simulink model "KillerWhaleModelPneumaticControl"  (R2020b)
settings: Solver=ode15s  StartTime=0.0  StopTime=10  MaxStep=0.01  RelTol=1e-3
model workspace: external: MATLAB File KillerWhaleParams.m (data not in the file)
undefined symbols (not defined in the file or in its folder): frontParams, rearParams, standParams, X, Y, Z
libraries: sm_lib x4301, nesl_utility x6
(part 3 of 66)

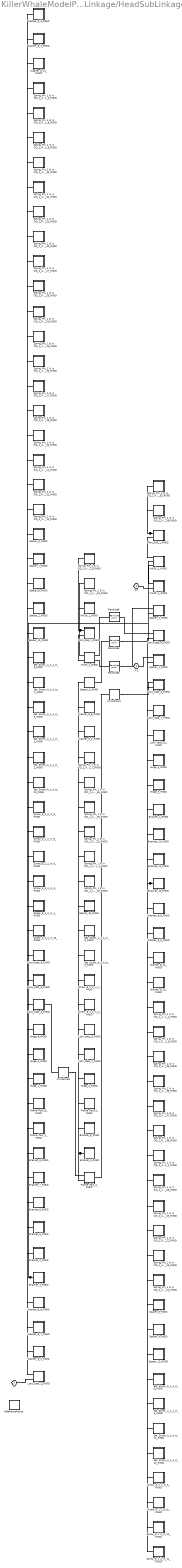
== system KillerWhaleModelPneumaticControl/HeadLinkage/HeadSubLinkage_1 ==
  Bracket_10_RIGID : Subsystem
  Bracket_11_RIGID : Subsystem
  Bracket_12_RIGID : Subsystem
  Bracket_1_RIGID : Subsystem
  Bracket_2_RIGID : Subsystem
  Bracket_3_RIGID : Subsystem
  Bracket_4_RIGID : Subsystem
  Bracket_5_RIGID : Subsystem
  Bracket_6_RIGID : Subsystem
  Bracket_7_RIGID : Subsystem
  Bracket_8_RIGID : Subsystem
  Bracket_9_RIGID : Subsystem
  Cylindrical1 : sm_lib/Joints/Cylindrical Joint  JointMode=Normal  SenseConstraintForce=off  SenseConstraintForceX=off  SenseConstraintForceY=off  SenseConstraintForceZ=off  SenseConstraintTorque=off  SenseConstraintTorqueX=off  SenseConstraintTorqueY=off  SenseConstraintTorqueZ=off  SenseTotalForce=off  SenseTotalForceX=off  SenseTotalForceY=off  SenseTotalForceZ=off  SenseTotalTorque=off  SenseTotalTorqueX=off  SenseTotalTorqueY=off  SenseTotalTorqueZ=off  CompositeWrenchDir=FollowerOnBase  CompositeWrenchFrame=BaseFrame  PzEquilibriumPosition=0  PzEquilibriumPositionUnits=m  PzSpringStiffness=0  PzSpringStiffnessUnits=N/m  PzDampingCoefficient=0  PzDampingCoefficientUnits=N/(m/s)  PzTorqueActuationMode=NoTorque  PzMotionActuationMode=ComputedMotion  PzSensePosition=off  PzSenseVelocity=off  PzSenseAcceleration=off  PzSenseTorqueForce=off  PzSenseLowerLimitTorqueForce=off  PzSenseUpperLimitTorqueForce=off  PzLowerLimitSpecify=off  PzLowerLimitBound=-1  PzLowerLimitBoundUnits=m  PzLowerLimitStiffness=1e6  PzLowerLimitStiffnessUnits=N/m  PzLowerLimitDamping=1e3  PzLowerLimitDampingUnits=N/(m/s)  PzLowerLimitTransitionRegionWidth=1e-4  PzLowerLimitTransitionRegionWidthUnits=m  PzUpperLimitSpecify=off  PzUpperLimitBound=1  PzUpperLimitBoundUnits=m  PzUpperLimitStiffness=1e6  PzUpperLimitStiffnessUnits=N/m  PzUpperLimitDamping=1e3  PzUpperLimitDampingUnits=N/(m/s)  PzUpperLimitTransitionRegionWidth=1e-4  PzUpperLimitTransitionRegionWidthUnits=m  PzPositionTargetSpecify=off  PzPositionTargetPriority=High  PzPositionTargetValue=0  PzPositionTargetValueUnits=m  PzVelocityTargetSpecify=off  PzVelocityTargetPriority=High  PzVelocityTargetValue=0  PzVelocityTargetValueUnits=m/s  RzEquilibriumPosition=0  RzEquilibriumPositionUnits=deg  RzSpringStiffness=0  RzSpringStiffnessUnits=N*m/deg  RzDampingCoefficient=0  RzDampingCoefficientUnits=N*m/(deg/s)  RzTorqueActuationMode=NoTorque  RzMotionActuationMode=ComputedMotion  RzSensePosition=off  RzSenseVelocity=off  RzSenseAcceleration=off  RzSenseTorqueForce=off  RzSenseLowerLimitTorqueForce=off  RzSenseUpperLimitTorqueForce=off  RzLowerLimitSpecify=off  RzLowerLimitBound=-90  RzLowerLimitBoundUnits=deg  RzLowerLimitStiffness=1e4  RzLowerLimitStiffnessUnits=N*m/deg  RzLowerLimitDamping=10  RzLowerLimitDampingUnits=N*m/(deg/s)  RzLowerLimitTransitionRegionWidth=0.1  RzLowerLimitTransitionRegionWidthUnits=deg  RzUpperLimitSpecify=off  RzUpperLimitBound=90  RzUpperLimitBoundUnits=deg  RzUpperLimitStiffness=1e4  RzUpperLimitStiffnessUnits=N*m/deg  RzUpperLimitDamping=10  RzUpperLimitDampingUnits=N*m/(deg/s)  RzUpperLimitTransitionRegionWidth=0.1  RzUpperLimitTransitionRegionWidthUnits=deg  RzPositionTargetSpecify=off  RzPositionTargetPriority=High  RzPositionTargetValue=0  RzPositionTargetValueUnits=deg  RzVelocityTargetSpecify=off  RzVelocityTargetPriority=High  RzVelocityTargetValue=0  RzVelocityTargetValueUnits=deg/s
  Cylindrical2 : sm_lib/Joints/Cylindrical Joint  JointMode=Normal  SenseConstraintForce=off  SenseConstraintForceX=off  SenseConstraintForceY=off  SenseConstraintForceZ=off  SenseConstraintTorque=off  SenseConstraintTorqueX=off  SenseConstraintTorqueY=off  SenseConstraintTorqueZ=off  SenseTotalForce=off  SenseTotalForceX=off  SenseTotalForceY=off  SenseTotalForceZ=off  SenseTotalTorque=off  SenseTotalTorqueX=off  SenseTotalTorqueY=off  SenseTotalTorqueZ=off  CompositeWrenchDir=FollowerOnBase  CompositeWrenchFrame=BaseFrame  PzEquilibriumPosition=0  PzEquilibriumPositionUnits=m  PzSpringStiffness=0  PzSpringStiffnessUnits=N/m  PzDampingCoefficient=0  PzDampingCoefficientUnits=N/(m/s)  PzTorqueActuationMode=NoTorque  PzMotionActuationMode=ComputedMotion  PzSensePosition=off  PzSenseVelocity=off  PzSenseAcceleration=off  PzSenseTorqueForce=off  PzSenseLowerLimitTorqueForce=off  PzSenseUpperLimitTorqueForce=off  PzLowerLimitSpecify=off  PzLowerLimitBound=-1  PzLowerLimitBoundUnits=m  PzLowerLimitStiffness=1e6  PzLowerLimitStiffnessUnits=N/m  PzLowerLimitDamping=1e3  PzLowerLimitDampingUnits=N/(m/s)  PzLowerLimitTransitionRegionWidth=1e-4  PzLowerLimitTransitionRegionWidthUnits=m  PzUpperLimitSpecify=off  PzUpperLimitBound=1  PzUpperLimitBoundUnits=m  PzUpperLimitStiffness=1e6  PzUpperLimitStiffnessUnits=N/m  PzUpperLimitDamping=1e3  PzUpperLimitDampingUnits=N/(m/s)  PzUpperLimitTransitionRegionWidth=1e-4  PzUpperLimitTransitionRegionWidthUnits=m  PzPositionTargetSpecify=off  PzPositionTargetPriority=High  PzPositionTargetValue=0  PzPositionTargetValueUnits=m  PzVelocityTargetSpecify=off  PzVelocityTargetPriority=High  PzVelocityTargetValue=0  PzVelocityTargetValueUnits=m/s  RzEquilibriumPosition=0  RzEquilibriumPositionUnits=deg  RzSpringStiffness=0  RzSpringStiffnessUnits=N*m/deg  RzDampingCoefficient=0  RzDampingCoefficientUnits=N*m/(deg/s)  RzTorqueActuationMode=NoTorque  RzMotionActuationMode=ComputedMotion  RzSensePosition=off  RzSenseVelocity=off  RzSenseAcceleration=off  RzSenseTorqueForce=off  RzSenseLowerLimitTorqueForce=off  RzSenseUpperLimitTorqueForce=off  RzLowerLimitSpecify=off  RzLowerLimitBound=-90  RzLowerLimitBoundUnits=deg  RzLowerLimitStiffness=1e4  RzLowerLimitStiffnessUnits=N*m/deg  RzLowerLimitDamping=10  RzLowerLimitDampingUnits=N*m/(deg/s)  RzLowerLimitTransitionRegionWidth=0.1  RzLowerLimitTransitionRegionWidthUnits=deg  RzUpperLimitSpecify=off  RzUpperLimitBound=90  RzUpperLimitBoundUnits=deg  RzUpperLimitStiffness=1e4  RzUpperLimitStiffnessUnits=N*m/deg  RzUpperLimitDamping=10  RzUpperLimitDampingUnits=N*m/(deg/s)  RzUpperLimitTransitionRegionWidth=0.1  RzUpperLimitTransitionRegionWidthUnits=deg  RzPositionTargetSpecify=off  RzPositionTargetPriority=High  RzPositionTargetValue=0  RzPositionTargetValueUnits=deg  RzVelocityTargetSpecify=off  RzVelocityTargetPriority=High  RzVelocityTargetValue=0  RzVelocityTargetValueUnits=deg/s
  Frame_Part_1_RIGID : Subsystem
  Frame_Part_2_RIGID : Subsystem
  Frame_Part_3_RIGID : Subsystem
  Frame_Part_4_RIGID : Subsystem
  Hinge_1_RIGID : Subsystem
  Hinge_2_RIGID : Subsystem
  Hinge_3_RIGID : Subsystem
  Hinge_4_RIGID : Subsystem
  Hinge_5_RIGID : Subsystem
  Hinge_6_RIGID : Subsystem
  Lock_tabs_10_RIGID : Subsystem
  Lock_tabs_1_RIGID : Subsystem
  Lock_tabs_2_RIGID : Subsystem
  Lock_tabs_3_RIGID : Subsystem
  Lock_tabs_4_RIGID : Subsystem
  Lock_tabs_5_RIGID : Subsystem
  Lock_tabs_6_RIGID : Subsystem
  Lock_tabs_7_RIGID : Subsystem
  Lock_tabs_8_RIGID : Subsystem
  Lock_tabs_9_RIGID : Subsystem
  Part_843_1_RIGID : Subsystem
  Part_844_1_RIGID : Subsystem
  ReferenceFrame : sm_lib/Frames and Transforms/Reference Frame
  Revolute3 : sm_lib/Joints/Revolute Joint  JointMode=Normal  SenseConstraintForce=off  SenseConstraintForceX=off  SenseConstraintForceY=off  SenseConstraintForceZ=off  SenseConstraintTorque=off  SenseConstraintTorqueX=off  SenseConstraintTorqueY=off  SenseConstraintTorqueZ=off  SenseTotalForce=off  SenseTotalForceX=off  SenseTotalForceY=off  SenseTotalForceZ=off  SenseTotalTorque=off  SenseTotalTorqueX=off  SenseTotalTorqueY=off  SenseTotalTorqueZ=off  CompositeWrenchDir=FollowerOnBase  CompositeWrenchFrame=BaseFrame  EquilibriumPosition=0  EquilibriumPositionUnits=deg  SpringStiffness=0  SpringStiffnessUnits=N*m/deg  DampingCoefficient=0  DampingCoefficientUnits=N*m/(deg/s)  TorqueActuationMode=NoTorque  MotionActuationMode=ComputedMotion  SensePosition=off  SenseVelocity=off  SenseAcceleration=off  SenseTorqueForce=off  SenseLowerLimitTorqueForce=off  SenseUpperLimitTorqueForce=off  LowerLimitSpecify=off  LowerLimitBound=-90  LowerLimitBoundUnits=deg  LowerLimitStiffness=1e4  LowerLimitStiffnessUnits=N*m/deg  LowerLimitDamping=10  LowerLimitDampingUnits=N*m/(deg/s)  LowerLimitTransitionRegionWidth=0.1  LowerLimitTransitionRegionWidthUnits=deg  UpperLimitSpecify=off  UpperLimitBound=90  UpperLimitBoundUnits=deg  UpperLimitStiffness=1e4  UpperLimitStiffnessUnits=N*m/deg  UpperLimitDamping=10  UpperLimitDampingUnits=N*m/(deg/s)  UpperLimitTransitionRegionWidth=0.1  UpperLimitTransitionRegionWidthUnits=deg  PositionTargetSpecify=on  PositionTargetPriority=Low  PositionTargetValue=frontParams.RevoluteJoint(3).Rz.Pos  PositionTargetValueUnits=deg  VelocityTargetSpecify=off  VelocityTargetPriority=High  VelocityTargetValue=0  VelocityTargetValueUnits=deg/s
  Revolute5 : sm_lib/Joints/Revolute Joint  JointMode=Normal  SenseConstraintForce=off  SenseConstraintForceX=off  SenseConstraintForceY=off  SenseConstraintForceZ=off  SenseConstraintTorque=off  SenseConstraintTorqueX=off  SenseConstraintTorqueY=off  SenseConstraintTorqueZ=off  SenseTotalForce=off  SenseTotalForceX=off  SenseTotalForceY=off  SenseTotalForceZ=off  SenseTotalTorque=off  SenseTotalTorqueX=off  SenseTotalTorqueY=off  SenseTotalTorqueZ=off  CompositeWrenchDir=FollowerOnBase  CompositeWrenchFrame=BaseFrame  EquilibriumPosition=0  EquilibriumPositionUnits=deg  SpringStiffness=0  SpringStiffnessUnits=N*m/deg  DampingCoefficient=0  DampingCoefficientUnits=N*m/(deg/s)  TorqueActuationMode=NoTorque  MotionActuationMode=ComputedMotion  SensePosition=off  SenseVelocity=off  SenseAcceleration=off  SenseTorqueForce=off  SenseLowerLimitTorqueForce=off  SenseUpperLimitTorqueForce=off  LowerLimitSpecify=off  LowerLimitBound=-90  LowerLimitBoundUnits=deg  LowerLimitStiffness=1e4  LowerLimitStiffnessUnits=N*m/deg  LowerLimitDamping=10  LowerLimitDampingUnits=N*m/(deg/s)  LowerLimitTransitionRegionWidth=0.1  LowerLimitTransitionRegionWidthUnits=deg  UpperLimitSpecify=off  UpperLimitBound=90  UpperLimitBoundUnits=deg  UpperLimitStiffness=1e4  UpperLimitStiffnessUnits=N*m/deg  UpperLimitDamping=10  UpperLimitDampingUnits=N*m/(deg/s)  UpperLimitTransitionRegionWidth=0.1  UpperLimitTransitionRegionWidthUnits=deg  PositionTargetSpecify=on  PositionTargetPriority=Low  PositionTargetValue=frontParams.RevoluteJoint(1).Rz.Pos  PositionTargetValueUnits=deg  VelocityTargetSpecify=off  VelocityTargetPriority=High  VelocityTargetValue=0  VelocityTargetValueUnits=deg/s
  Revolute6 : sm_lib/Joints/Revolute Joint  JointMode=Normal  SenseConstraintForce=off  SenseConstraintForceX=off  SenseConstraintForceY=off  SenseConstraintForceZ=off  SenseConstraintTorque=off  SenseConstraintTorqueX=off  SenseConstraintTorqueY=off  SenseConstraintTorqueZ=off  SenseTotalForce=off  SenseTotalForceX=off  SenseTotalForceY=off  SenseTotalForceZ=off  SenseTotalTorque=off  SenseTotalTorqueX=off  SenseTotalTorqueY=off  SenseTotalTorqueZ=off  CompositeWrenchDir=FollowerOnBase  CompositeWrenchFrame=BaseFrame  EquilibriumPosition=0  EquilibriumPositionUnits=deg  SpringStiffness=0  SpringStiffnessUnits=N*m/deg  DampingCoefficient=0  DampingCoefficientUnits=N*m/(deg/s)  TorqueActuationMode=NoTorque  MotionActuationMode=ComputedMotion  SensePosition=off  SenseVelocity=off  SenseAcceleration=off  SenseTorqueForce=off  SenseLowerLimitTorqueForce=off  SenseUpperLimitTorqueForce=off  LowerLimitSpecify=off  LowerLimitBound=-90  LowerLimitBoundUnits=deg  LowerLimitStiffness=1e4  LowerLimitStiffnessUnits=N*m/deg  LowerLimitDamping=10  LowerLimitDampingUnits=N*m/(deg/s)  LowerLimitTransitionRegionWidth=0.1  LowerLimitTransitionRegionWidthUnits=deg  UpperLimitSpecify=off  UpperLimitBound=90  UpperLimitBoundUnits=deg  UpperLimitStiffness=1e4  UpperLimitStiffnessUnits=N*m/deg  UpperLimitDamping=10  UpperLimitDampingUnits=N*m/(deg/s)  UpperLimitTransitionRegionWidth=0.1  UpperLimitTransitionRegionWidthUnits=deg  PositionTargetSpecify=on  PositionTargetPriority=Low  PositionTargetValue=frontParams.RevoluteJoint(2).Rz.Pos  PositionTargetValueUnits=deg  VelocityTargetSpecify=off  VelocityTargetPriority=High  VelocityTargetValue=0  VelocityTargetValueUnits=deg/s
  Screw_8_1_2_in_10_RIGID : Subsystem
  Screw_8_1_2_in_11_RIGID : Subsystem
  Screw_8_1_2_in_12_RIGID : Subsystem
  Screw_8_1_2_in_1_RIGID : Subsystem
  Screw_8_1_2_in_2_RIGID : Subsystem
  Screw_8_1_2_in_3_RIGID : Subsystem
  Screw_8_1_2_in_4_RIGID : Subsystem
  Screw_8_1_2_in_5_RIGID : Subsystem
  Screw_8_1_2_in_6_RIGID : Subsystem
  Screw_8_1_2_in_7_RIGID : Subsystem
  Screw_8_1_2_in_8_RIGID : Subsystem
  Screw_8_1_2_in_9_RIGID : Subsystem
  Set_Screw_4_1_4_in_10_RIGID : Subsystem
  Set_Screw_4_1_4_in_11_RIGID : Subsystem
  Set_Screw_4_1_4_in_12_RIGID : Subsystem
  Set_Screw_4_1_4_in_1_RIGID : Subsystem
  Set_Screw_4_1_4_in_2_RIGID : Subsystem
  Set_Screw_4_1_4_in_3_RIGID : Subsystem
  Set_Screw_4_1_4_in_4_RIGID : Subsystem
  Set_Screw_4_1_4_in_5_RIGID : Subsystem
  Set_Screw_4_1_4_in_6_RIGID : Subsystem
  Set_Screw_4_1_4_in_7_RIGID : Subsystem
  Set_Screw_4_1_4_in_8_RIGID : Subsystem
  Set_Screw_4_1_4_in_9_RIGID : Subsystem
  Spacer_10_RIGID : Subsystem
  Spacer_11_RIGID : Subsystem
  Spacer_12_RIGID : Subsystem
  Spacer_1_RIGID : Subsystem
  Spacer_2_RIGID : Subsystem
  Spacer_3_RIGID : Subsystem
  Spacer_4_RIGID : Subsystem
  Spacer_5_RIGID : Subsystem
  Spacer_6_RIGID : Subsystem
  Spacer_7_RIGID : Subsystem
  Spacer_8_RIGID : Subsystem
  Spacer_9_RIGID : Subsystem
  Spring_Pin_1_8_in_OD_1_4_in_L_10_RIGID : Subsystem
  Spring_Pin_1_8_in_OD_1_4_in_L_11_RIGID : Subsystem
  Spring_Pin_1_8_in_OD_1_4_in_L_12_RIGID : Subsystem
  Spring_Pin_1_8_in_OD_1_4_in_L_13_RIGID : Subsystem
  Spring_Pin_1_8_in_OD_1_4_in_L_14_RIGID : Subsystem
  Spring_Pin_1_8_in_OD_1_4_in_L_15_RIGID : Subsystem
  Spring_Pin_1_8_in_OD_1_4_in_L_16_RIGID : Subsystem
  Spring_Pin_1_8_in_OD_1_4_in_L_17_RIGID : Subsystem
  Spring_Pin_1_8_in_OD_1_4_in_L_18_RIGID : Subsystem
  Spring_Pin_1_8_in_OD_1_4_in_L_19_RIGID : Subsystem
  Spring_Pin_1_8_in_OD_1_4_in_L_1_RIGID : Subsystem
  Spring_Pin_1_8_in_OD_1_4_in_L_20_RIGID : Subsystem
  Spring_Pin_1_8_in_OD_1_4_in_L_21_RIGID : Subsystem
  Spring_Pin_1_8_in_OD_1_4_in_L_22_RIGID : Subsystem
  Spring_Pin_1_8_in_OD_1_4_in_L_23_RIGID : Subsystem
  Spring_Pin_1_8_in_OD_1_4_in_L_24_RIGID : Subsystem
  Spring_Pin_1_8_in_OD_1_4_in_L_25_RIGID : Subsystem
  Spring_Pin_1_8_in_OD_1_4_in_L_26_RIGID : Subsystem
  Spring_Pin_1_8_in_OD_1_4_in_L_27_RIGID : Subsystem
  Spring_Pin_1_8_in_OD_1_4_in_L_28_RIGID : Subsystem
  Spring_Pin_1_8_in_OD_1_4_in_L_29_RIGID : Subsystem
  Spring_Pin_1_8_in_OD_1_4_in_L_2_RIGID : Subsystem
  Spring_Pin_1_8_in_OD_1_4_in_L_30_RIGID : Subsystem
  Spring_Pin_1_8_in_OD_1_4_in_L_31_RIGID : Subsystem
  Spring_Pin_1_8_in_OD_1_4_in_L_32_RIGID : Subsystem
  Spring_Pin_1_8_in_OD_1_4_in_L_33_RIGID : Subsystem
  Spring_Pin_1_8_in_OD_1_4_in_L_34_RIGID : Subsystem
  Spring_Pin_1_8_in_OD_1_4_in_L_35_RIGID : Subsystem
  Spring_Pin_1_8_in_OD_1_4_in_L_36_RIGID : Subsystem
  Spring_Pin_1_8_in_OD_1_4_in_L_37_RIGID : Subsystem
  Spring_Pin_1_8_in_OD_1_4_in_L_38_RIGID : Subsystem
  Spring_Pin_1_8_in_OD_1_4_in_L_39_RIGID : Subsystem
  Spring_Pin_1_8_in_OD_1_4_in_L_3_RIGID : Subsystem
  Spring_Pin_1_8_in_OD_1_4_in_L_40_RIGID : Subsystem
  Spring_Pin_1_8_in_OD_1_4_in_L_4_RIGID : Subsystem
  Spring_Pin_1_8_in_OD_1_4_in_L_5_RIGID : Subsystem
  Spring_Pin_1_8_in_OD_1_4_in_L_6_RIGID : Subsystem
  Spring_Pin_1_8_in_OD_1_4_in_L_7_RIGID : Subsystem
  Spring_Pin_1_8_in_OD_1_4_in_L_8_RIGID : Subsystem
  Spring_Pin_1_8_in_OD_1_4_in_L_9_RIGID : Subsystem
  Washer_8_10_RIGID : Subsystem
  Washer_8_11_RIGID : Subsystem
  Washer_8_12_RIGID : Subsystem
  Washer_8_1_RIGID : Subsystem
  Washer_8_2_RIGID : Subsystem
  Washer_8_3_RIGID : Subsystem
  Washer_8_4_RIGID : Subsystem
  Washer_8_5_RIGID : Subsystem
  Washer_8_6_RIGID : Subsystem
  Washer_8_7_RIGID : Subsystem
  Washer_8_8_RIGID : Subsystem
  Washer_8_9_RIGID : Subsystem
  link1fl_1_RIGID : Subsystem
  link1fr_1_RIGID : Subsystem
  link2fl_1_RIGID : Subsystem
  link2fr_1_RIGID : Subsystem
  F2 : PMIOPort  Side=Left
  F1 : PMIOPort  Port=2  Side=Left
  F : PMIOPort  Port=3  Side=Right
  connections:
  Bracket_1_RIGID/LConn1 -- Bracket_2_RIGID/LConn1 -- Bracket_5_RIGID/LConn1 -- Bracket_6_RIGID/LConn1 -- Bracket_7_RIGID/LConn1 -- Bracket_9_RIGID/LConn1 -- Frame_Part_1_RIGID/LConn1 -- Frame_Part_3_RIGID/LConn1 -- Hinge_1_RIGID/LConn1 -- Hinge_5_RIGID/LConn1 -- Hinge_6_RIGID/LConn1 -- Lock_tabs_1_RIGID/LConn1 -- Lock_tabs_3_RIGID/LConn1 -- Lock_tabs_8_RIGID/LConn1 -- Lock_tabs_9_RIGID/LConn1 -- Screw_8_1_2_in_10_RIGID/LConn1 -- Screw_8_1_2_in_1_RIGID/LConn1 -- Screw_8_1_2_in_3_RIGID/LConn1 -- Screw_8_1_2_in_4_RIGID/LConn1 -- Screw_8_1_2_in_8_RIGID/LConn1 -- Screw_8_1_2_in_9_RIGID/LConn1 -- Set_Screw_4_1_4_in_12_RIGID/LConn1 -- Set_Screw_4_1_4_in_1_RIGID/LConn1 -- Set_Screw_4_1_4_in_2_RIGID/LConn1 -- Set_Screw_4_1_4_in_6_RIGID/LConn1 -- Set_Screw_4_1_4_in_7_RIGID/LConn1 -- Set_Screw_4_1_4_in_8_RIGID/LConn1 -- Spacer_11_RIGID/LConn1 -- Spacer_2_RIGID/LConn1 -- Spacer_5_RIGID/LConn2 -- Spacer_6_RIGID/LConn1 -- Spacer_7_RIGID/LConn1 -- Spacer_9_RIGID/LConn1 -- Spring_Pin_1_8_in_OD_1_4_in_L_11_RIGID/LConn1 -- Spring_Pin_1_8_in_OD_1_4_in_L_12_RIGID/LConn1 -- Spring_Pin_1_8_in_OD_1_4_in_L_14_RIGID/LConn1 -- Spring_Pin_1_8_in_OD_1_4_in_L_15_RIGID/LConn1 -- Spring_Pin_1_8_in_OD_1_4_in_L_16_RIGID/LConn1 -- Spring_Pin_1_8_in_OD_1_4_in_L_17_RIGID/LConn1 -- Spring_Pin_1_8_in_OD_1_4_in_L_20_RIGID/LConn1 -- Spring_Pin_1_8_in_OD_1_4_in_L_23_RIGID/LConn1 -- Spring_Pin_1_8_in_OD_1_4_in_L_24_RIGID/LConn1 -- Spring_Pin_1_8_in_OD_1_4_in_L_26_RIGID/LConn1 -- Spring_Pin_1_8_in_OD_1_4_in_L_27_RIGID/LConn1 -- Spring_Pin_1_8_in_OD_1_4_in_L_30_RIGID/LConn1 -- Spring_Pin_1_8_in_OD_1_4_in_L_31_RIGID/LConn1 -- Spring_Pin_1_8_in_OD_1_4_in_L_32_RIGID/LConn1 -- Spring_Pin_1_8_in_OD_1_4_in_L_40_RIGID/LConn1 -- Spring_Pin_1_8_in_OD_1_4_in_L_6_RIGID/LConn1 -- Spring_Pin_1_8_in_OD_1_4_in_L_8_RIGID/LConn1 -- Spring_Pin_1_8_in_OD_1_4_in_L_9_RIGID/LConn1 -- Washer_8_11_RIGID/LConn1 -- Washer_8_1_RIGID/LConn1 -- Washer_8_3_RIGID/LConn1 -- Washer_8_4_RIGID/LConn1 -- Washer_8_7_RIGID/LConn1 -- Washer_8_9_RIGID/LConn1
  Bracket_10_RIGID/LConn1 -- Bracket_11_RIGID/LConn1 -- Bracket_12_RIGID/LConn1 -- Bracket_4_RIGID/LConn1 -- Hinge_3_RIGID/LConn1 -- Hinge_4_RIGID/LConn1 -- Lock_tabs_10_RIGID/LConn1 -- Lock_tabs_4_RIGID/LConn2 -- Lock_tabs_5_RIGID/LConn2 -- Lock_tabs_7_RIGID/LConn1 -- Screw_8_1_2_in_11_RIGID/LConn1 -- Screw_8_1_2_in_12_RIGID/LConn1 -- Screw_8_1_2_in_5_RIGID/LConn1 -- Screw_8_1_2_in_6_RIGID/LConn1 -- Set_Screw_4_1_4_in_10_RIGID/LConn1 -- Set_Screw_4_1_4_in_11_RIGID/LConn1 -- Set_Screw_4_1_4_in_4_RIGID/LConn1 -- Set_Screw_4_1_4_in_5_RIGID/LConn1 -- Spacer_12_RIGID/LConn1 -- Spacer_1_RIGID/LConn2 -- Spacer_4_RIGID/LConn1 -- Spacer_8_RIGID/LConn1 -- Spring_Pin_1_8_in_OD_1_4_in_L_10_RIGID/LConn1 -- Spring_Pin_1_8_in_OD_1_4_in_L_13_RIGID/LConn1 -- Spring_Pin_1_8_in_OD_1_4_in_L_22_RIGID/LConn1 -- Spring_Pin_1_8_in_OD_1_4_in_L_25_RIGID/LConn1 -- Spring_Pin_1_8_in_OD_1_4_in_L_28_RIGID/LConn1 -- Spring_Pin_1_8_in_OD_1_4_in_L_2_RIGID/LConn1 -- Spring_Pin_1_8_in_OD_1_4_in_L_36_RIGID/LConn1 -- Spring_Pin_1_8_in_OD_1_4_in_L_37_RIGID/LConn1 -- Spring_Pin_1_8_in_OD_1_4_in_L_38_RIGID/LConn1 -- Spring_Pin_1_8_in_OD_1_4_in_L_39_RIGID/LConn1 -- Spring_Pin_1_8_in_OD_1_4_in_L_3_RIGID/LConn1 -- Spring_Pin_1_8_in_OD_1_4_in_L_4_RIGID/LConn1 -- Washer_8_10_RIGID/LConn1 -- Washer_8_12_RIGID/LConn1 -- Washer_8_5_RIGID/LConn1 -- Washer_8_6_RIGID/LConn1
  Revolute5/RConn1 -- Spacer_5_RIGID/LConn1
  Revolute6/LConn1 -- link2fl_1_RIGID/RConn1
  Lock_tabs_4_RIGID/LConn1 -- Revolute6/RConn1
  Cylindrical2/LConn1 -- Lock_tabs_3_RIGID/RConn1
  Cylindrical2/RConn1 -- Frame_Part_2_RIGID/LConn1
  Part_844_1_RIGID/LConn2 -- link2fl_1_RIGID/LConn2
  Revolute3/LConn1 -- Spacer_3_RIGID/RConn1
  Revolute3/RConn1 -- link1fl_1_RIGID/LConn3
  Part_843_1_RIGID/LConn2 -- link1fl_1_RIGID/LConn1
  Lock_tabs_1_RIGID/LConn2 -- F/RConn1
  link1fl_1_RIGID/LConn2 -- link1fr_1_RIGID/LConn1
  Spacer_1_RIGID/LConn1 -- F1/RConn1
  link1fr_1_RIGID/LConn2 -- F2/RConn1
  Part_843_1_RIGID/LConn1 -- Spring_Pin_1_8_in_OD_1_4_in_L_18_RIGID/LConn1 -- Spring_Pin_1_8_in_OD_1_4_in_L_33_RIGID/LConn1
  link2fl_1_RIGID/LConn1 -- link2fr_1_RIGID/LConn1
  Bracket_3_RIGID/LConn1 -- Bracket_8_RIGID/LConn1 -- Frame_Part_2_RIGID/LConn2 -- Frame_Part_4_RIGID/LConn1 -- Hinge_2_RIGID/LConn1 -- Lock_tabs_2_RIGID/LConn1 -- Lock_tabs_6_RIGID/LConn1 -- Screw_8_1_2_in_2_RIGID/LConn1 -- Screw_8_1_2_in_7_RIGID/LConn1 -- Set_Screw_4_1_4_in_3_RIGID/LConn1 -- Set_Screw_4_1_4_in_9_RIGID/LConn1 -- Spacer_10_RIGID/LConn1 -- Spacer_3_RIGID/LConn1 -- Spring_Pin_1_8_in_OD_1_4_in_L_19_RIGID/LConn1 -- Spring_Pin_1_8_in_OD_1_4_in_L_1_RIGID/LConn1 -- Spring_Pin_1_8_in_OD_1_4_in_L_21_RIGID/LConn1 -- Spring_Pin_1_8_in_OD_1_4_in_L_29_RIGID/LConn1 -- Spring_Pin_1_8_in_OD_1_4_in_L_35_RIGID/LConn1 -- Spring_Pin_1_8_in_OD_1_4_in_L_7_RIGID/LConn1 -- Washer_8_2_RIGID/LConn1 -- Washer_8_8_RIGID/LConn1
  Part_844_1_RIGID/LConn1 -- Spring_Pin_1_8_in_OD_1_4_in_L_34_RIGID/LConn1 -- Spring_Pin_1_8_in_OD_1_4_in_L_5_RIGID/LConn1
  Cylindrical1/LConn1 -- Frame_Part_2_RIGID/RConn1
  Cylindrical1/RConn1 -- Lock_tabs_5_RIGID/LConn1
  Revolute5/LConn1 -- link2fl_1_RIGID/RConn2

== system KillerWhaleModelPneumaticControl/HeadLinkage/Head_Actuator_1 ==
  Part_10_1_RIGID : Subsystem
  Part_11_1_RIGID : Subsystem
  Part_12_1_RIGID : Subsystem
  Part_13_1_RIGID : Subsystem
  Part_1_1_RIGID : Subsystem
  Part_2_1_RIGID : Subsystem
  Part_3_1_RIGID : Subsystem
  Part_4_1_RIGID : Subsystem
  Part_5_1_RIGID : Subsystem
  Part_6_1_RIGID : Subsystem
  Part_7_1_RIGID : Subsystem
  Part_8_1_RIGID : Subsystem
  Part_9_1_RIGID : Subsystem
  ReferenceFrame : sm_lib/Frames and Transforms/Reference Frame
  Slider1 : sm_lib/Joints/Prismatic Joint  JointMode=Normal  SenseConstraintForce=off  SenseConstraintForceX=off  SenseConstraintForceY=off  SenseConstraintForceZ=off  SenseConstraintTorque=off  SenseConstraintTorqueX=off  SenseConstraintTorqueY=off  SenseConstraintTorqueZ=off  SenseTotalForce=off  SenseTotalForceX=off  SenseTotalForceY=off  SenseTotalForceZ=off  SenseTotalTorque=off  SenseTotalTorqueX=off  SenseTotalTorqueY=off  SenseTotalTorqueZ=off  CompositeWrenchDir=FollowerOnBase  CompositeWrenchFrame=BaseFrame  EquilibriumPosition=0  EquilibriumPositionUnits=m  SpringStiffness=0  SpringStiffnessUnits=N/m  DampingCoefficient=0  DampingCoefficientUnits=N/(m/s)  TorqueActuationMode=ComputedTorque  MotionActuationMode=InputMotion  SensePosition=off  SenseVelocity=off  SenseAcceleration=off  SenseTorqueForce=off  SenseLowerLimitTorqueForce=off  SenseUpperLimitTorqueForce=off  LowerLimitSpecify=off  LowerLimitBound=-1  LowerLimitBoundUnits=m  LowerLimitStiffness=1e6  LowerLimitStiffnessUnits=N/m  LowerLimitDamping=1e3  LowerLimitDampingUnits=N/(m/s)  LowerLimitTransitionRegionWidth=1e-4  LowerLimitTransitionRegionWidthUnits=m  UpperLimitSpecify=off  UpperLimitBound=1  UpperLimitBoundUnits=m  UpperLimitStiffness=1e6  UpperLimitStiffnessUnits=N/m  UpperLimitDamping=1e3  UpperLimitDampingUnits=N/(m/s)  UpperLimitTransitionRegionWidth=1e-4  UpperLimitTransitionRegionWidthUnits=m  PositionTargetSpecify=on  PositionTargetPriority=Low  PositionTargetValue=frontParams.PrismaticJoint(2).Pz.Pos  PositionTargetValueUnits=in  VelocityTargetSpecify=off  VelocityTargetPriority=High  VelocityTargetValue=0  VelocityTargetValueUnits=m/s
  Transform : sm_lib/Frames and Transforms/Rigid Transform  TranslationMethod=Cartesian  TranslationStandardOffset=0  TranslationLengthUnit=in  TranslationStandardAxis=+Z  TranslationCartesianOffset=frontParams.RigidTransform(421).translation  TranslationROffset=0  TranslationROffsetUnits=m  TranslationZOffset=0  TranslationZOffsetUnits=m  TranslationThetaOffset=0  TranslationThetaOffsetUnits=deg  RotationMethod=ArbitraryAxis  RotationAngleUnits=rad  RotationStandardAxis=+Z  RotationAngle=frontParams.RigidTransform(421).angle  RotationArbitraryAxis=frontParams.RigidTransform(421).axis  FollAlignAxisA=+X  BaseAlignAxisA=+Y  FollAlignAxisB=+Y  BaseAlignAxisB=+Z  RotationSequenceAxes=FollowerAxes  RotationSequence=XYX  RotationSequenceAngles=[0 0 0]  RotationSequenceAnglesUnits=deg  RotationMatrix=[1 0 0; 0 1 0; 0 0 1]
  F : PMIOPort  Side=Left
  F1 : PMIOPort  Port=2  Side=Right
  J4 : PMIOPort  Port=3  Side=Right
  connections:
  Part_10_1_RIGID/LConn1 -- Part_5_1_RIGID/LConn2 -- Part_7_1_RIGID/LConn1 -- Part_6_1_RIGID/LConn1 -- Part_4_1_RIGID/LConn1 -- Part_12_1_RIGID/LConn1 -- Part_8_1_RIGID/LConn1
  Part_11_1_RIGID/LConn1 -- Part_2_1_RIGID/LConn1 -- Part_9_1_RIGID/LConn1 -- Part_3_1_RIGID/LConn1 -- Part_13_1_RIGID/LConn1 -- Part_1_1_RIGID/LConn2
  Part_4_1_RIGID/RConn1 -- Slider1/LConn1
  Part_9_1_RIGID/LConn2 -- Slider1/RConn1
  Part_10_1_RIGID/LConn2 -- F/RConn1
  Part_1_1_RIGID/LConn1 -- F1/RConn1
  Part_5_1_RIGID/LConn1 -- Transform/RConn1
  ReferenceFrame/RConn1 -- Transform/LConn1
  J4/RConn1 -- Slider1/LConn2

== system KillerWhaleModelPneumaticControl/HeadLinkage/Neck_Actuator_1 ==
  Part_14_1_RIGID : Subsystem
  Part_15_1_RIGID : Subsystem
  Part_16_1_RIGID : Subsystem
  Part_17_1_RIGID : Subsystem
  Part_18_1_RIGID : Subsystem
  Part_19_1_RIGID : Subsystem
  Part_20_1_RIGID : Subsystem
  Part_21_1_RIGID : Subsystem
  Part_22_1_RIGID : Subsystem
  Part_23_1_RIGID : Subsystem
  Part_24_1_RIGID : Subsystem
  Part_25_1_RIGID : Subsystem
  Part_26_1_RIGID : Subsystem
  ReferenceFrame : sm_lib/Frames and Transforms/Reference Frame
  Slider1 : sm_lib/Joints/Prismatic Joint  JointMode=Normal  SenseConstraintForce=off  SenseConstraintForceX=off  SenseConstraintForceY=off  SenseConstraintForceZ=off  SenseConstraintTorque=off  SenseConstraintTorqueX=off  SenseConstraintTorqueY=off  SenseConstraintTorqueZ=off  SenseTotalForce=off  SenseTotalForceX=off  SenseTotalForceY=off  SenseTotalForceZ=off  SenseTotalTorque=off  SenseTotalTorqueX=off  SenseTotalTorqueY=off  SenseTotalTorqueZ=off  CompositeWrenchDir=FollowerOnBase  CompositeWrenchFrame=BaseFrame  EquilibriumPosition=0  EquilibriumPositionUnits=m  SpringStiffness=0  SpringStiffnessUnits=N/m  DampingCoefficient=0  DampingCoefficientUnits=N/(m/s)  TorqueActuationMode=ComputedTorque  MotionActuationMode=InputMotion  SensePosition=off  SenseVelocity=off  SenseAcceleration=off  SenseTorqueForce=off  SenseLowerLimitTorqueForce=off  SenseUpperLimitTorqueForce=off  LowerLimitSpecify=off  LowerLimitBound=-1  LowerLimitBoundUnits=m  LowerLimitStiffness=1e6  LowerLimitStiffnessUnits=N/m  LowerLimitDamping=1e3  LowerLimitDampingUnits=N/(m/s)  LowerLimitTransitionRegionWidth=1e-4  LowerLimitTransitionRegionWidthUnits=m  UpperLimitSpecify=off  UpperLimitBound=1  UpperLimitBoundUnits=m  UpperLimitStiffness=1e6  UpperLimitStiffnessUnits=N/m  UpperLimitDamping=1e3  UpperLimitDampingUnits=N/(m/s)  UpperLimitTransitionRegionWidth=1e-4  UpperLimitTransitionRegionWidthUnits=m  PositionTargetSpecify=on  PositionTargetPriority=Low  PositionTargetValue=frontParams.PrismaticJoint(1).Pz.Pos  PositionTargetValueUnits=in  VelocityTargetSpecify=off  VelocityTargetPriority=High  VelocityTargetValue=0  VelocityTargetValueUnits=m/s
  Transform : sm_lib/Frames and Transforms/Rigid Transform  TranslationMethod=Cartesian  TranslationStandardOffset=0  TranslationLengthUnit=in  TranslationStandardAxis=+Z  TranslationCartesianOffset=frontParams.RigidTransform(420).translation  TranslationROffset=0  TranslationROffsetUnits=m  TranslationZOffset=0  TranslationZOffsetUnits=m  TranslationThetaOffset=0  TranslationThetaOffsetUnits=deg  RotationMethod=ArbitraryAxis  RotationAngleUnits=rad  RotationStandardAxis=+Z  RotationAngle=frontParams.RigidTransform(420).angle  RotationArbitraryAxis=frontParams.RigidTransform(420).axis  FollAlignAxisA=+X  BaseAlignAxisA=+Y  FollAlignAxisB=+Y  BaseAlignAxisB=+Z  RotationSequenceAxes=FollowerAxes  RotationSequence=XYX  RotationSequenceAngles=[0 0 0]  RotationSequenceAnglesUnits=deg  RotationMatrix=[1 0 0; 0 1 0; 0 0 1]
  F : PMIOPort  Side=Left
  J3 : PMIOPort  Port=2  Side=Left
  F1 : PMIOPort  Port=3  Side=Right
  connections:
  Part_14_1_RIGID/LConn1 -- Part_16_1_RIGID/LConn1 -- Part_25_1_RIGID/LConn1 -- Part_23_1_RIGID/LConn2 -- Part_26_1_RIGID/LConn2 -- Part_15_1_RIGID/LConn1
  Part_17_1_RIGID/LConn1 -- Part_21_1_RIGID/LConn1 -- Part_22_1_RIGID/LConn1 -- Part_20_1_RIGID/LConn1 -- Part_19_1_RIGID/LConn1 -- Part_24_1_RIGID/LConn1 -- Part_18_1_RIGID/LConn2
  Part_17_1_RIGID/RConn1 -- Slider1/LConn1
  Part_26_1_RIGID/LConn1 -- Slider1/RConn1
  Part_23_1_RIGID/LConn1 -- F/RConn1
  Part_17_1_RIGID/LConn2 -- F1/RConn1
  Part_18_1_RIGID/LConn1 -- Transform/RConn1
  ReferenceFrame/RConn1 -- Transform/LConn1
  J3/RConn1 -- Slider1/LConn2

== system KillerWhaleModelPneumaticControl/RearLinkage/Tail_Actuator_1_1 ==
  Part_40_1_RIGID : Subsystem
  Part_41_1_RIGID : Subsystem
  Part_42_1_RIGID : Subsystem
  Part_43_1_RIGID : Subsystem
  Part_44_1_RIGID : Subsystem
  Part_45_1_RIGID : Subsystem
  Part_46_1_RIGID : Subsystem
  Part_47_1_RIGID : Subsystem
  Part_48_1_RIGID : Subsystem
  Part_49_1_RIGID : Subsystem
  Part_50_1_RIGID : Subsystem
  Part_51_1_RIGID : Subsystem
  Part_52_1_RIGID : Subsystem
  ReferenceFrame : sm_lib/Frames and Transforms/Reference Frame
  Slider1 : sm_lib/Joints/Prismatic Joint  JointMode=Normal  SenseConstraintForce=off  SenseConstraintForceX=off  SenseConstraintForceY=off  SenseConstraintForceZ=off  SenseConstraintTorque=off  SenseConstraintTorqueX=off  SenseConstraintTorqueY=off  SenseConstraintTorqueZ=off  SenseTotalForce=off  SenseTotalForceX=off  SenseTotalForceY=off  SenseTotalForceZ=off  SenseTotalTorque=off  SenseTotalTorqueX=off  SenseTotalTorqueY=off  SenseTotalTorqueZ=off  CompositeWrenchDir=FollowerOnBase  CompositeWrenchFrame=BaseFrame  EquilibriumPosition=0  EquilibriumPositionUnits=m  SpringStiffness=0  SpringStiffnessUnits=N/m  DampingCoefficient=0  DampingCoefficientUnits=N/(m/s)  TorqueActuationMode=ComputedTorque  MotionActuationMode=InputMotion  SensePosition=off  SenseVelocity=off  SenseAcceleration=off  SenseTorqueForce=off  SenseLowerLimitTorqueForce=off  SenseUpperLimitTorqueForce=off  LowerLimitSpecify=off  LowerLimitBound=-1  LowerLimitBoundUnits=m  LowerLimitStiffness=1e6  LowerLimitStiffnessUnits=N/m  LowerLimitDamping=1e3  LowerLimitDampingUnits=N/(m/s)  LowerLimitTransitionRegionWidth=1e-4  LowerLimitTransitionRegionWidthUnits=m  UpperLimitSpecify=off  UpperLimitBound=1  UpperLimitBoundUnits=m  UpperLimitStiffness=1e6  UpperLimitStiffnessUnits=N/m  UpperLimitDamping=1e3  UpperLimitDampingUnits=N/(m/s)  UpperLimitTransitionRegionWidth=1e-4  UpperLimitTransitionRegionWidthUnits=m  PositionTargetSpecify=on  PositionTargetPriority=Low  PositionTargetValue=rearParams.PrismaticJoint(1).Pz.Pos  PositionTargetValueUnits=in  VelocityTargetSpecify=off  VelocityTargetPriority=High  VelocityTargetValue=0  VelocityTargetValueUnits=m/s
  Transform : sm_lib/Frames and Transforms/Rigid Transform  TranslationMethod=Cartesian  TranslationStandardOffset=0  TranslationLengthUnit=in  TranslationStandardAxis=+Z  TranslationCartesianOffset=rearParams.RigidTransform(787).translation  TranslationROffset=0  TranslationROffsetUnits=m  TranslationZOffset=0  TranslationZOffsetUnits=m  TranslationThetaOffset=0  TranslationThetaOffsetUnits=deg  RotationMethod=ArbitraryAxis  RotationAngleUnits=rad  RotationStandardAxis=+Z  RotationAngle=rearParams.RigidTransform(787).angle  RotationArbitraryAxis=rearParams.RigidTransform(787).axis  FollAlignAxisA=+X  BaseAlignAxisA=+Y  FollAlignAxisB=+Y  BaseAlignAxisB=+Z  RotationSequenceAxes=FollowerAxes  RotationSequence=XYX  RotationSequenceAngles=[0 0 0]  RotationSequenceAnglesUnits=deg  RotationMatrix=[1 0 0; 0 1 0; 0 0 1]
  J2 : PMIOPort  Side=Left
  F1 : PMIOPort  Port=2  Side=Right
  F : PMIOPort  Port=3  Side=Right
  connections:
  Part_41_1_RIGID/LConn1 -- Part_42_1_RIGID/LConn1 -- Part_52_1_RIGID/LConn2 -- Part_40_1_RIGID/LConn1 -- Part_49_1_RIGID/LConn1 -- Part_51_1_RIGID/LConn1
  Part_44_1_RIGID/LConn2 -- Part_43_1_RIGID/LConn1 -- Part_47_1_RIGID/LConn1 -- Part_48_1_RIGID/LConn1 -- Part_46_1_RIGID/LConn1 -- Part_45_1_RIGID/LConn1 -- Part_50_1_RIGID/LConn1
  Part_43_1_RIGID/RConn1 -- Slider1/LConn1
  Part_52_1_RIGID/LConn1 -- Slider1/RConn1
  Part_43_1_RIGID/LConn2 -- F/RConn1
  Part_40_1_RIGID/LConn2 -- F1/RConn1
  Part_44_1_RIGID/LConn1 -- Transform/RConn1
  ReferenceFrame/RConn1 -- Transform/LConn1
  J2/RConn1 -- Slider1/LConn2

== system KillerWhaleModelPneumaticControl/RearLinkage/Tail_Actuator_2_1 ==
  Part_27_1_RIGID : Subsystem
  Part_28_1_RIGID : Subsystem
  Part_29_1_RIGID : Subsystem
  Part_30_1_RIGID : Subsystem
  Part_31_1_RIGID : Subsystem
  Part_32_1_RIGID : Subsystem
  Part_33_1_RIGID : Subsystem
  Part_34_1_RIGID : Subsystem
  Part_35_1_RIGID : Subsystem
  Part_36_1_RIGID : Subsystem
  Part_37_1_RIGID : Subsystem
  Part_38_1_RIGID : Subsystem
  Part_39_1_RIGID : Subsystem
  ReferenceFrame : sm_lib/Frames and Transforms/Reference Frame
  Slider1 : sm_lib/Joints/Prismatic Joint  JointMode=Normal  SenseConstraintForce=off  SenseConstraintForceX=off  SenseConstraintForceY=off  SenseConstraintForceZ=off  SenseConstraintTorque=off  SenseConstraintTorqueX=off  SenseConstraintTorqueY=off  SenseConstraintTorqueZ=off  SenseTotalForce=off  SenseTotalForceX=off  SenseTotalForceY=off  SenseTotalForceZ=off  SenseTotalTorque=off  SenseTotalTorqueX=off  SenseTotalTorqueY=off  SenseTotalTorqueZ=off  CompositeWrenchDir=FollowerOnBase  CompositeWrenchFrame=BaseFrame  EquilibriumPosition=0  EquilibriumPositionUnits=m  SpringStiffness=0  SpringStiffnessUnits=N/m  DampingCoefficient=0  DampingCoefficientUnits=N/(m/s)  TorqueActuationMode=ComputedTorque  MotionActuationMode=InputMotion  SensePosition=off  SenseVelocity=off  SenseAcceleration=off  SenseTorqueForce=off  SenseLowerLimitTorqueForce=off  SenseUpperLimitTorqueForce=off  LowerLimitSpecify=off  LowerLimitBound=-1  LowerLimitBoundUnits=m  LowerLimitStiffness=1e6  LowerLimitStiffnessUnits=N/m  LowerLimitDamping=1e3  LowerLimitDampingUnits=N/(m/s)  LowerLimitTransitionRegionWidth=1e-4  LowerLimitTransitionRegionWidthUnits=m  UpperLimitSpecify=off  UpperLimitBound=1  UpperLimitBoundUnits=m  UpperLimitStiffness=1e6  UpperLimitStiffnessUnits=N/m  UpperLimitDamping=1e3  UpperLimitDampingUnits=N/(m/s)  UpperLimitTransitionRegionWidth=1e-4  UpperLimitTransitionRegionWidthUnits=m  PositionTargetSpecify=on  PositionTargetPriority=Low  PositionTargetValue=rearParams.PrismaticJoint(2).Pz.Pos  PositionTargetValueUnits=in  VelocityTargetSpecify=off  VelocityTargetPriority=High  VelocityTargetValue=0  VelocityTargetValueUnits=m/s
  Transform : sm_lib/Frames and Transforms/Rigid Transform  TranslationMethod=Cartesian  TranslationStandardOffset=0  TranslationLengthUnit=in  TranslationStandardAxis=+Z  TranslationCartesianOffset=rearParams.RigidTransform(788).translation  TranslationROffset=0  TranslationROffsetUnits=m  TranslationZOffset=0  TranslationZOffsetUnits=m  TranslationThetaOffset=0  TranslationThetaOffsetUnits=deg  RotationMethod=ArbitraryAxis  RotationAngleUnits=rad  RotationStandardAxis=+Z  RotationAngle=rearParams.RigidTransform(788).angle  RotationArbitraryAxis=rearParams.RigidTransform(788).axis  FollAlignAxisA=+X  BaseAlignAxisA=+Y  FollAlignAxisB=+Y  BaseAlignAxisB=+Z  RotationSequenceAxes=FollowerAxes  RotationSequence=XYX  RotationSequenceAngles=[0 0 0]  RotationSequenceAnglesUnits=deg  RotationMatrix=[1 0 0; 0 1 0; 0 0 1]
  J1 : PMIOPort  Side=Left
  F1 : PMIOPort  Port=2  Side=Right
  F : PMIOPort  Port=3  Side=Right
  connections:
  Part_30_1_RIGID/LConn2 -- Part_29_1_RIGID/LConn1 -- Part_33_1_RIGID/LConn1 -- Part_34_1_RIGID/LConn1 -- Part_32_1_RIGID/LConn1 -- Part_31_1_RIGID/LConn1 -- Part_36_1_RIGID/LConn1
  Part_28_1_RIGID/LConn1 -- Part_38_1_RIGID/LConn2 -- Part_39_1_RIGID/LConn2 -- Part_27_1_RIGID/LConn1 -- Part_35_1_RIGID/LConn1 -- Part_37_1_RIGID/LConn1
  Part_29_1_RIGID/RConn1 -- Slider1/LConn1
  Part_38_1_RIGID/LConn1 -- Slider1/RConn1
  Part_29_1_RIGID/LConn2 -- F/RConn1
  Part_39_1_RIGID/LConn1 -- F1/RConn1
  Part_30_1_RIGID/LConn1 -- Transform/RConn1
  ReferenceFrame/RConn1 -- Transform/LConn1
  J1/RConn1 -- Slider1/LConn2
